simulink model "test_filter"  (R2021a)
settings: Solver=VariableStepAuto  StartTime=0.0  StopTime=5  RelTol=1e-3
libraries: Butterworth x2, simulink x1, dspfdesign x1
settings Model: Creator=ge26jow  LastModifiedBy=ge26jow

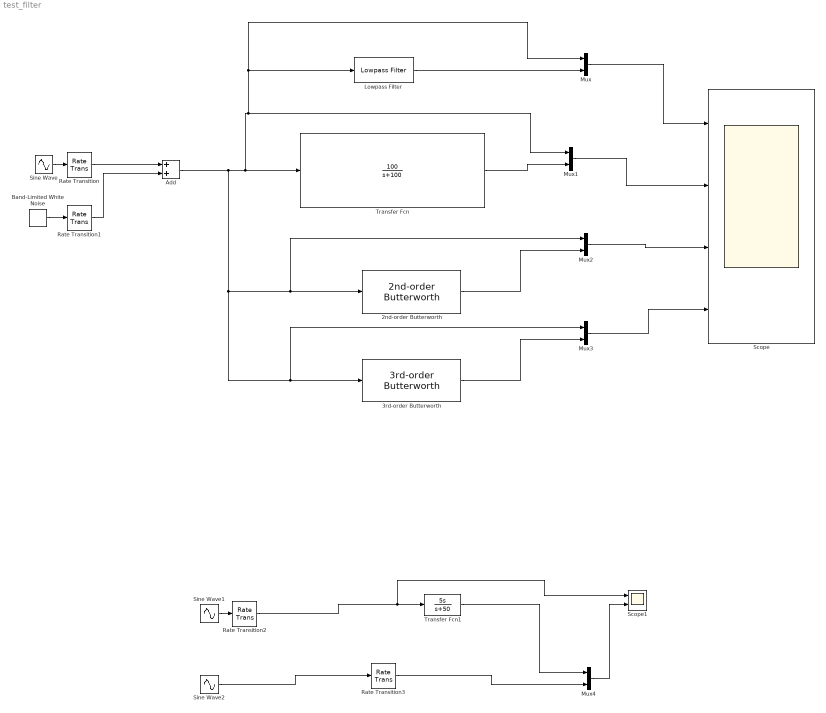
== system test_filter ==
  2nd-order Butterworth : Butterworth/2nd-order Butterworth  Gain=1  omegac=100
  3rd-order Butterworth : Butterworth/3rd-order Butterworth  Gain=1  omegac=100
  Add : Sum
  Band-Limited White Noise : simulink/Sources/Band-Limited White Noise  Cov=[1e-5]  Ts=1e-3  seed=[23341]
  Lowpass Filter : dspfdesign/Lowpass Filter  FilterType=FIR  DesignForMinimumOrder=on  FilterOrder=50  PassbandFrequency=300  StopbandFrequency=400  PassbandRipple=0.1  StopbandAttenuation=80  InheritSampleRate=on  SampleRate=44100  SimulateUsing=Interpreted execution  roundingMode=Floor  coeffsDataTypeStr=fixdt(1,16)
  Mux{,1..4} (5 alike) : Mux  Inputs=2
  Rate Transition{,1..3} (4 alike) : RateTransition  OutPortSampleTime=1e-3
  Scope : Scope  NumInputPorts=4
  Scope1 : Scope  NumInputPorts=2
  Sine Wave : Sin  Frequency=10  SampleTime=1e-4
  Sine Wave1 : Sin  Frequency=10  SampleTime=1e-4
  Sine Wave2 : Sin  Frequency=10  Phase=pi/2  SampleTime=1e-4
  Transfer Fcn : TransferFcn  Numerator=[100]  Denominator=[1 100]
  Transfer Fcn1 : TransferFcn  Numerator=[5 0]  Denominator=[1 50]
  wires:
  Lowpass Filter/1 -> Mux/2
  Transfer Fcn/1 -> Mux1/2
  Mux1/1 -> Scope/2
  Mux/1 -> Scope/1
  Sine Wave/1 -> Rate Transition/1
  Band-Limited White Noise/1 -> Rate Transition1/1
  2nd-order Butterworth/1 -> Mux2/2
  Mux2/1 -> Scope/3
  3rd-order Butterworth/1 -> Mux3/2
  Add/1 -> Mux3/1, 3rd-order Butterworth/1, Mux2/1, 2nd-order Butterworth/1, Lowpass Filter/1, Mux/1, Mux1/1, Transfer Fcn/1
  Mux3/1 -> Scope/4
  Rate Transition/1 -> Add/1
  Rate Transition1/1 -> Add/2
  Rate Transition2/1 -> Scope1/1, Transfer Fcn1/1
  Sine Wave1/1 -> Rate Transition2/1
  Rate Transition3/1 -> Mux4/2
  Sine Wave2/1 -> Rate Transition3/1
  Transfer Fcn1/1 -> Mux4/1
  Mux4/1 -> Scope1/2
